simulink model "adc"  (Simulink 8.7)
settings: Solver=ode45  StartTime=0.0  StopTime=1000  RelTol=1e-3
settings Model: Creator=33105  LastModifiedBy=33105
settings DataIOCC: LimitDataPoints=off  SaveFormat=Dataset
settings DebuggingCC: UnderspecifiedInitializationDetection=Simplified  MergeDetectMultiDrivingBlocksExec=error
settings HardwareCC: ProdBitPerPointer=64  ProdLargestAtomicFloat=Float  ProdIntDivRoundTo=Zero  ProdEndianess=LittleEndian  ProdWordSize=64  ProdHWDeviceType=Intel->x86-64 (Windows64)
settings ModelReferenceCC: PropagateSignalLabelsOutOfModel=on
settings ConfigComp: CovModelRefEnable=off

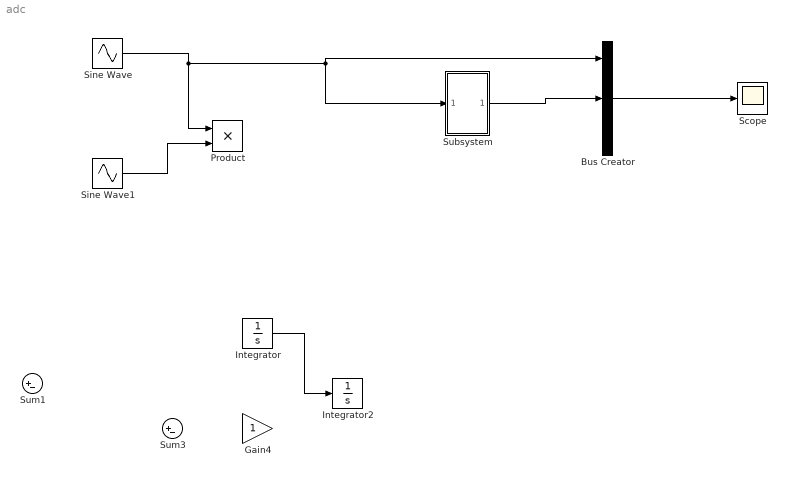
== system adc ==
  Bus Creator : BusCreator  Inputs=3
  Gain4 : Gain
  Integrator : Integrator
  Integrator2 : Integrator
  Product : Product
  Scope : Scope
  Sine Wave : Sin  SampleTime=0
  Sine Wave1 : Sin  SampleTime=0
  Subsystem : Subsystem
  Sum1 : Sum  Inputs=|+-
  Sum3 : Sum  Inputs=|+-
  wires:
  Integrator/1 -> Integrator2/1
  Sine Wave/1 -> Subsystem/1(In1), Bus Creator/1, Product/1
  Sine Wave1/1 -> Product/2
  Bus Creator/1 -> Scope/1
  Subsystem/1(Out1) -> Bus Creator/2

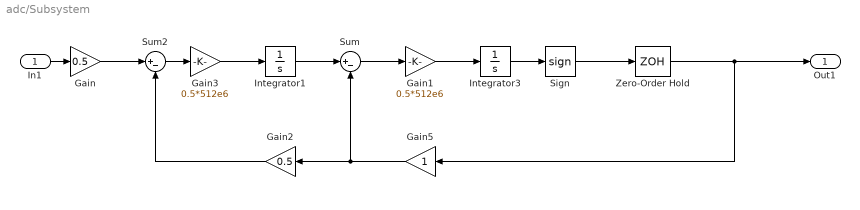
== system adc/Subsystem ==
  In1 : Inport
  Gain : Gain  Gain=0.5
  Gain1 : Gain  Gain=0.5*512e6
  Gain2 : Gain  Gain=0.5
  Gain3 : Gain  Gain=0.5*512e6
  Gain5 : Gain
  Integrator1 : Integrator
  Integrator3 : Integrator
  Sign : Signum
  Sum : Sum  Inputs=|+-
  Sum2 : Sum  Inputs=|+-
  Zero-Order Hold : ZeroOrderHold
  Out1 : Outport
  wires:
  In1/1 -> Gain/1
  Gain/1 -> Sum2/1
  Sum2/1 -> Gain3/1
  Sign/1 -> Zero-Order Hold/1
  Zero-Order Hold/1 -> Out1/1, Gain5/1
  Gain3/1 -> Integrator1/1
  Gain5/1 -> Gain2/1, Sum/2
  Integrator1/1 -> Sum/1
  Sum/1 -> Gain1/1
  Gain1/1 -> Integrator3/1
  Integrator3/1 -> Sign/1
  Gain2/1 -> Sum2/2
